simulink model "RefAdjSup"  (R2025b)
settings: Solver=ode14x  StartTime=0.0  StopTime=10.0  FixedStep=Ts_local  RelTol=1e-3
model workspace (MAT data in the model file):
  FSI_max = [111.58614649; 109.244229433; 111.951462771]
  FSI_min = [3.65502707696; 3.64264743495; 3.42913459589]
  K1 = 1
  K2 = 1e-06
  Ncycle = 25
  SampEn_max = [0.399850516102; 0.373441099122; 0.45958437331]
  SampEn_min = [0.118794892672; 0.117721768048; 0.119599512992]
  fs = 5000
  m = 2
  rRatio = 0.2
values from neighbouring files (symbols this model uses):
  f = 50.0    [ctrlSys.sldd]
  Ts_ctrl = 0.1    [ctrlSys.sldd]
  Ts_local = 1.0E-5    [ctrlSys.sldd]
libraries: fuzblock x3
settings Model: DataDictionary=ctrlSys.sldd  Creator=i336  LastModifiedBy=i336

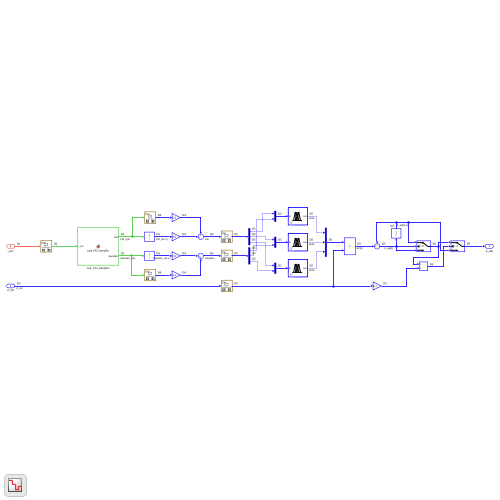
[thumbnail: Simulink's stored preview of the top-level diagram]
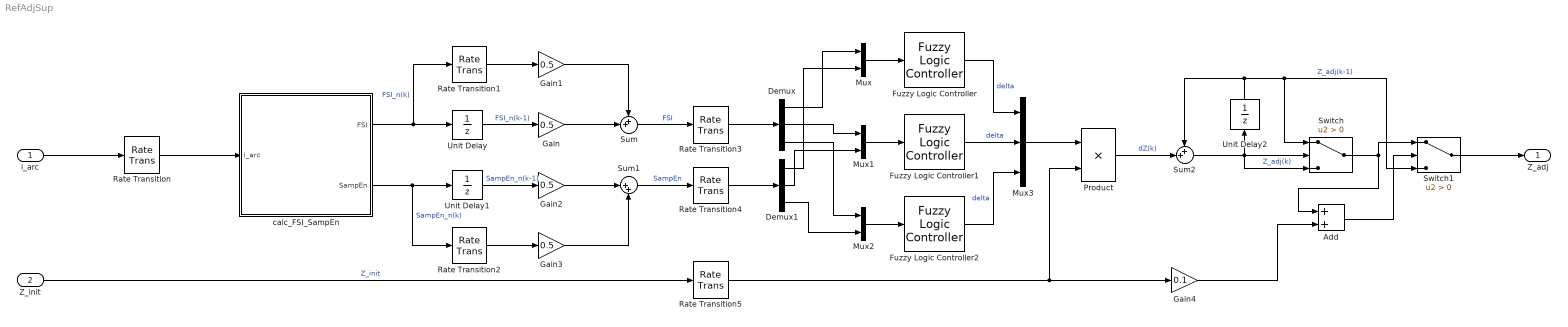
== system RefAdjSup ==
  i_arc : Inport  SampleTime=Ts_local
  Z_init : Inport  Port=2  PortDimensions=[3 1]  SampleTime=Ts_ctrl
  Add : Sum
  Demux : Demux  Outputs=3
  Demux1 : Demux  Outputs=3
  Fuzzy Logic Controller : fuzblock/Fuzzy Logic  Controller  FIS=fis  OutputSampleNumber=101  DataType=double  UseLookupTable=off  NumBreakpoints=10  FuzzifiedInputs=off  RuleFiringStrengths=off  RuleOutputs=off  AggregatedOutputs=off  SimulateUsing=Interpreted execution  OutOfRangeInputValueMessage=warning  NoRuleFiredMessage=warning  EmptyOutputFuzzySetMessage=warning
  Fuzzy Logic Controller1 : fuzblock/Fuzzy Logic  Controller  FIS=fis  OutputSampleNumber=101  DataType=double  UseLookupTable=off  NumBreakpoints=10  FuzzifiedInputs=off  RuleFiringStrengths=off  RuleOutputs=off  AggregatedOutputs=off  SimulateUsing=Interpreted execution  OutOfRangeInputValueMessage=warning  NoRuleFiredMessage=warning  EmptyOutputFuzzySetMessage=warning
  Fuzzy Logic Controller2 : fuzblock/Fuzzy Logic  Controller  FIS=fis  OutputSampleNumber=101  DataType=double  UseLookupTable=off  NumBreakpoints=10  FuzzifiedInputs=off  RuleFiringStrengths=off  RuleOutputs=off  AggregatedOutputs=off  SimulateUsing=Interpreted execution  OutOfRangeInputValueMessage=warning  NoRuleFiredMessage=warning  EmptyOutputFuzzySetMessage=warning
  Gain{,1..3} (4 alike) : Gain  Gain=0.5
  Gain4 : Gain  Gain=0.1
  Mux : Mux  Inputs=2
  Mux1 : Mux  Inputs=2
  Mux2 : Mux  Inputs=2
  Mux3 : Mux  Inputs=3
  Product : Product
  Rate Transition : RateTransition  OutPortSampleTime=1 / fs
  Rate Transition1 : RateTransition  OutPortSampleTime=Ncycle * (1 / f)
  Rate Transition2 : RateTransition  OutPortSampleTime=Ncycle * (1 / f)
  Rate Transition3 : RateTransition  OutPortSampleTime=Ts_sup
  Rate Transition4 : RateTransition  OutPortSampleTime=Ts_sup
  Rate Transition5 : RateTransition  OutPortSampleTime=Ts_sup
  Sum : Sum  Inputs=++|
  Sum1 : Sum  Inputs=|++
  Sum2 : Sum  Inputs=++|
  Switch : Switch  Criteria=u2 > Threshold  SaturateOnIntegerOverflow=off  InputSameDT=off
  Switch1 : Switch  Criteria=u2 > Threshold  SaturateOnIntegerOverflow=off  InputSameDT=off
  Unit Delay : UnitDelay  SampleTime=Ncycle * (1 / f)  HasFrameUpgradeWarning=on
  Unit Delay1 : UnitDelay  SampleTime=Ncycle * (1 / f)  HasFrameUpgradeWarning=on
  Unit Delay2 : UnitDelay  SampleTime=-1  HasFrameUpgradeWarning=on
  calc_FSI_SampEn : MATLAB Function  TreatAsAtomicUnit=on  SystemSampleTime=1 / fs
  Z_adj : Outport
  wires:
  i_arc/1 -> Rate Transition/1
  Rate Transition/1 -> calc_FSI_SampEn/1(i_arc)
  calc_FSI_SampEn/1(FSI) -> Rate Transition1/1, Unit Delay/1  "FSI_n(k)"
  calc_FSI_SampEn/2(SampEn) -> Rate Transition2/1, Unit Delay1/1  "SampEn_n(k)"
  Unit Delay/1 -> Gain/1  "FSI_n(k-1)"
  Gain/1 -> Sum/2
  Gain1/1 -> Sum/1
  Gain2/1 -> Sum1/1
  Gain3/1 -> Sum1/2
  Unit Delay1/1 -> Gain2/1  "SampEn_n(k-1)"
  Rate Transition1/1 -> Gain1/1
  Rate Transition2/1 -> Gain3/1
  Z_init/1 -> Rate Transition5/1  "Z_init"
  Sum2/1 -> Switch/3, Switch/2, Unit Delay2/1  "Z_adj(k)"
  Mux/1 -> Fuzzy Logic Controller/1
  Mux2/1 -> Fuzzy Logic Controller2/1
  Mux1/1 -> Fuzzy Logic Controller1/1
  Demux/1 -> Mux/1
  Demux1/1 -> Mux/2
  Demux/2 -> Mux1/1
  Demux1/2 -> Mux1/2
  Demux/3 -> Mux2/1
  Demux1/3 -> Mux2/2
  Mux3/1 -> Product/1
  Fuzzy Logic Controller/1 -> Mux3/1  "delta"
  Fuzzy Logic Controller1/1 -> Mux3/2  "delta"
  Fuzzy Logic Controller2/1 -> Mux3/3  "delta"
  Sum/1 -> Rate Transition3/1  "FSI"
  Rate Transition3/1 -> Demux/1
  Sum1/1 -> Rate Transition4/1  "SampEn"
  Rate Transition4/1 -> Demux1/1
  Rate Transition5/1 -> Gain4/1, Product/2
  Unit Delay2/1 -> Sum2/1, Switch1/3, Switch/1  "Z_adj(k-1)"
  Product/1 -> Sum2/2  "dZ(k)"
  Gain4/1 -> Add/2
  Add/1 -> Switch1/2
  Switch/1 -> Add/1, Switch1/1
  Switch1/1 -> Z_adj/1

== matlab function RefAdjSup/calc_FSI_SampEn ==
  data: i_arc input size=[3 1]; FSI output; SampEn output; K1 parameter size=[1 1]; K2 parameter size=[1 1]; fs parameter size=[1 1]; Ncycle parameter size=[1 1]; f parameter size=[1 1]; m parameter size=[1 1]; rRatio parameter size=[1 1]; FSI_max parameter size=[3 1]; FSI_min parameter size=[3 1]; SampEn_max parameter size=[3 1]; SampEn_min parameter size=[3 1]
function [FSI, SampEn] = calc_FSI_SampEn( ...
    i_arc, K1, K2, fs, Ncycle, f, m, rRatio, ...
    FSI_max, FSI_min, SampEn_max, SampEn_min)
%#codegen
% i_arc   : 3x1 instantaneous arc current [ia; ib; ic]
% FSI     : 3x1 normalized FSI of three phases
% SampEn  : 3x1 normalized sample entropy of three phases
%
% This version:
% 1) stores samples every call,
% 2) computes features only once every Nhop samples,
% 3) holds the last computed outputs between updates.

    Nwin = int32(Ncycle * fs / f);   % assume exact integer
    Nhop = Nwin;                     % non-overlapping windows
    % For overlapped windows, e.g.:
    % Nhop = int32(Nwin/2);

    persistent buf head count sinceCalc lastFSI lastSampEn

    if isempty(head)
        buf        = zeros(Nwin, 3);
        head       = int32(0);
        count      = int32(0);
        sinceCalc  = int32(0);
        lastFSI    = zeros(3,1);
        lastSampEn = zeros(3,1);
    end

    % Ensure column vector
    i_arc = reshape(i_arc, 3, 1);

    % -------------------------
    % 1) Update circular buffer
    % -------------------------
    head = head + 1;
    if head > Nwin
        head = int32(1);
    end

    buf(head, :) = i_arc.';

    if count < Nwin
        count = count + 1;
    end

    sinceCalc = sinceCalc + 1;

    % Default outputs: hold last values
    FSI    = lastFSI;
    SampEn = lastSampEn;

    % Before first full window, output zeros
    if count < Nwin
        FSI(:)    = 0.0;
        SampEn(:) = 0.0;
        return;
    end

    % -----------------------------------------
    % 2) Only recompute once every Nhop samples
    % -----------------------------------------
    if sinceCalc < Nhop
        return;
    end
    sinceCalc = int32(0);

    % Reconstruct ordered window: oldest --> newest
    xwin = zeros(Nwin, 3);
    if head < Nwin
        n1 = Nwin - head;
        xwin(1:n1, :)      = buf(head+1:Nwin, :);
        xwin(n1+1:Nwin, :) = buf(1:head, :);
    else
        xwin = buf;
    end

    % Compute features phase by phase
    for p = 1:3
        x = xwin(:, p);

        fsi_raw = local_fsi(x, fs, f, K1, K2);
        den1 = FSI_max(p) - FSI_min(p);
        if abs(den1) <= 1e-12
            FSI(p) = 0.0;
        else
            FSI_n = (fsi_raw - FSI_min(p)) / den1;
            FSI(p) = min(max(FSI_n, 0.0), 1.0);
        end

        se_raw = local_sampen(x, m, rRatio);
        den2 = SampEn_max(p) - SampEn_min(p);
        if abs(den2) <= 1e-12
            SampEn(p) = 0.0;
        else
            SampEn_n = (se_raw - SampEn_min(p)) / den2;
            SampEn(p) = min(max(SampEn_n, 0.0), 1.0);
        end
    end

    % Save outputs for holding until next update
    lastFSI    = FSI;
    lastSampEn = SampEn;
end

function y = local_fsi(x, fs, f0, K1, K2)
% Compute FSI from one phase current window

    x = x(:);
    N = length(x);

    % Remove DC component
    x = x - mean(x);

    % FFT
    X = fft(x);

    % Single-sided amplitude spectrum
    nHalf = floor(N/2) + 1;
    A = 2.0 * abs(X(1:nHalf)) / N;
    A(1) = abs(X(1)) / N;
    if mod(N, 2) == 0
        A(end) = abs(X(nHalf)) / N;
    end

    % Extract harmonic amplitudes H1 ... H20
    H = zeros(20, 1);
    for h = 1:20
        k = round(h * f0 / fs * N) + 1;
        if k >= 1 && k <= nHalf
            H(h) = A(k);
        else
            H(h) = 0.0;
        end
    end

    denom = K1 * sqrt(sum(H(10:20).^2)) + K2;

    if denom <= 1e-12
        y = 0.0;
    else
        y = H(1) / denom;
    end
end

function se = local_sampen(x, m, rRatio)
% Compute sample entropy of one phase current window

    x = x(:);
    N = length(x);

    if N <= m + 1
        se = 0.0;
        return;
    end

    sigma = std(x);
    r = rRatio * sigma;

    if r <= 1e-12
        se = 0.0;
        return;
    end

    A = 0.0;
    B = 0.0;

    Nm = N - m;

    for i = 1:Nm
        for j = i+1:Nm
            match_m = true;

            for k = 0:m-1
                if abs(x(i+k) - x(j+k)) > r
                    match_m = false;
                    break;
                end
            end

            if match_m
                B = B + 1.0;

                if abs(x(i+m) - x(j+m)) <= r
                    A = A + 1.0;
                end
            end
        end
    end

    se = -log((A + realmin) / (B + realmin));
end
